simulink model "Mammalian_Model"  (R2020b)
settings: Solver=ode3  StartTime=t(1)  StopTime=t(end)  FixedStep=dt  RelTol=1e-3
values from neighbouring files (symbols this model uses):
  params = [ ... (first row only)    [gois09_simulink.m]    (also in ryzhii14_simulink.m; sinoatrial_simulink.m; vdp_simulink.m)
undefined symbols (not defined in the file or in its folder): y0
settings Model: Creator=chukw  LastModifiedBy=chukw

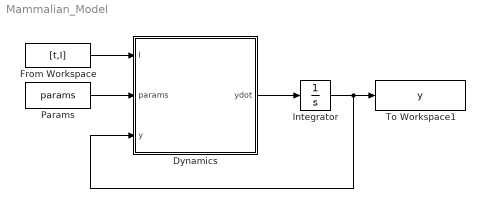
== system Mammalian_Model ==
  Dynamics : MATLAB Function  TreatAsAtomicUnit=on
  From Workspace : FromWorkspace  VariableName=[t,I]
  Integrator : Integrator  InitialCondition=y0
  Params : Constant  Value=params
  To Workspace1 : ToWorkspace  VariableName=y  SampleTime=-1
  wires:
  From Workspace/1 -> Dynamics/1(I)
  Integrator/1 -> Dynamics/3(y), To Workspace1/1
  Dynamics/1(ydot) -> Integrator/1
  Params/1 -> Dynamics/2(params)

== matlab function Mammalian_Model/Dynamics ==
  data: I input; params input; ydot output; y input
function ydot = dyn(I,params,y)
    v1b = params(1);
    k1b = params(2);
    kli = params(3);
    k1d = params(4);
    k2b = params(5);
    k2d = params(6);
    k3d = params(7);
    k2t = params(8);
    k3t = params(9);
    v4b = params(10);
    k4b = params(11);
    k4d = params(12);
    k5b = params(13);
    k5d = params(14);
    k5t = params(15);
    k6d = params(16);
    k6t = params(17);
    k6p = params(18);
    k7d = params(19);
    k7p = params(20);
    c = params(21);
    p = params(22);
    q = params(23);
    r = params(24);
    
    ydot = zeros(7,1);
    
    ydot(1) = ((v1b*(y(7) + c))/(k1b*(1 + (y(3)/kli)^p) + (y(7) + c))) -...
                k1d*y(1) + I;
    ydot(2) = k2b*(y(1)^q) - k2d*y(2) - k2t*y(2) + k3t*y(3);
    ydot(3) = k2t*y(2) - k3t*y(3) - k3d*y(3);
    ydot(4) = ((v4b*y(3)^r)/(k4b + y(3)^r)) - k4d*y(4);
    ydot(5) = k5b*y(4) - k5d*y(5) - k5t*y(5) + k6t*y(6);
    ydot(6) = k5t*y(5) - k6t*y(6) -k6d*y(6) + k7p*y(7) - k6p*y(6);
    ydot(7) = k6p*y(6) - k7p*y(7) - k7d*y(7);
end
